simulink model "continuous_control_4_1"  (R2021b)
settings: Solver=VariableStepAuto  StartTime=0.0  StopTime=10.0  RelTol=1e-3
values from neighbouring files (symbols this model uses):
  f1 = F(1)    [in_lab.m]
  f2 = F(2)    [in_lab.m]
  u_bar = sqrt(g*x_bar(1)^2)    [in_lab.m]    (also in prelab.m)
  x_bar = [0.5; 0.0]    [in_lab.m]    (also in prelab.m)
settings Model: Creator=pranshumalik14  LastModifiedBy=varunsampat
settings SolverCC: AlgebraicLoopSolver=TrustRegion
settings DataIOCC: ReturnWorkspaceOutputs=off
settings DebuggingCC: SFMachineParentedDataDiag=warning  ArithmeticOperatorsInVariantConditions=warning
settings SFSimCC: CustomCodeUndefinedFunction=UseInterfaceOnly

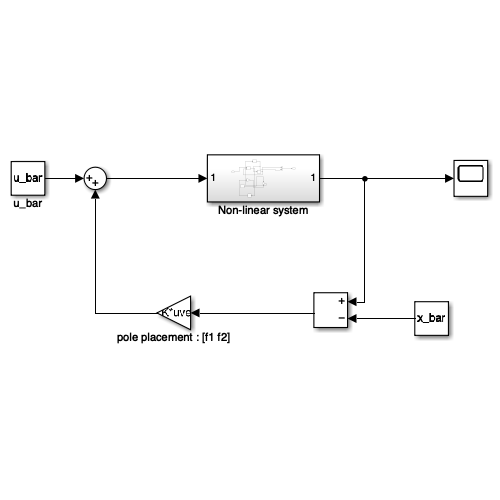
[thumbnail: Simulink's stored preview of the top-level diagram]
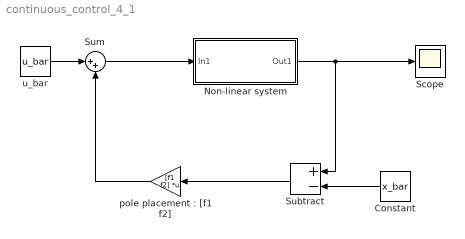
== system continuous_control_4_1 ==
  Constant : Constant  Value=x_bar
  Non-linear system : Subsystem
  Scope : Scope
  Subtract : Sum  Inputs=+-
  Sum : Sum  Inputs=|++
  "pole placement : [f1 f2]" : Gain  Gain=[f1 f2]  Multiplication=Matrix(K*u) (u vector)
  u_bar : Constant  Value=u_bar
  wires:
  Non-linear system/1(Out1) -> Subtract/1, Scope/1
  u_bar/1 -> Sum/1
  "pole placement : [f1 f2]"/1 -> Sum/2
  Sum/1 -> Non-linear system/1(In1)
  Constant/1 -> Subtract/2
  Subtract/1 -> "pole placement : [f1 f2]"/1

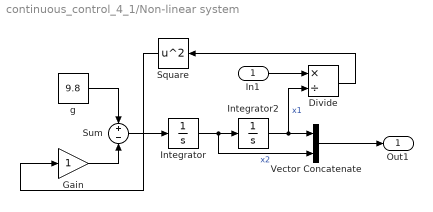
== system continuous_control_4_1/Non-linear system ==
  In1 : Inport
  Divide : Product  Inputs=*/
  Gain : Gain
  Integrator : Integrator  InitialCondition=0.5
  Integrator2 : Integrator  InitialCondition=1.3
  Square : Math  Operator=square  SignedPower=on  SaturateOnIntegerOverflow=on
  Sum : Sum  Inputs=+-
  Vector Concatenate : Concatenate
  g : Constant  Value=9.8
  Out1 : Outport  VectorParamsAs1DForOutWhenUnconnected=off
  wires:
  Integrator2/1 -> Vector Concatenate/1, Divide/2  "x1"
  In1/1 -> Divide/1
  g/1 -> Sum/1
  Sum/1 -> Integrator/1
  Square/1 -> Gain/1
  Divide/1 -> Square/1
  Gain/1 -> Sum/2
  Integrator/1 -> Vector Concatenate/2, Integrator2/1  "x2"
  Vector Concatenate/1 -> Out1/1
